simulink model "SimscapeCrane_StepInput"  (R2015a)
settings: Solver=ode15s  StartTime=0.0  StopTime=T  RelTol=1e-3
values from neighbouring files (symbols this model uses):
  filter_denominator = cell2mat(disc_filter.den)    [test.m]
  filter_numerator = cell2mat(disc_filter.num)    [test.m]
  H = B_big'*Q_big*B_big + R_big    [test.m]
  h_x = A_big'*Q_big*B_big    [test.m]
  m = 1    [test.m]
  N = 30    [test.m]
  Ts = 0.01    [test.m]
  Ts_mpc = 0.1    [test.m]
undefined symbols (not defined in the file or in its folder): MR, TxBreak, TxCoulomb, TxVisc, TyBreak, TyCoulomb, TzBreak, TzCoulomb, X, xRange, xZero, Y, yRange, yZero, Z, zRange, zZero
undefined symbols (not defined in the file): M, TorqueMultX, TorqueMultY, TorqueMultZ, TxTrans, TyTrans, TyVisc, TzTrans, TzVisc
libraries: sm_lib x146, fl_lib x62, nesl_utility x24, elec_lib x9, simulink x9, sm_double_wishbone_suspension_lib x4, aerolibtransform2 x1
(part 1 of 15)
settings Model: Creator=jsustare  LastModifiedBy=bkhusain
settings SolverCC: MaxConsecutiveMinStep=10  AutoInsertRateTranBlk=on  InsertRTBMode=Never (minimum delay)
settings DataIOCC: LimitDataPoints=off  SaveFormat=StructureWithTime
settings HardwareCC: ProdBitPerPointer=64  ProdLargestAtomicFloat=Float  ProdIntDivRoundTo=Zero  ProdEndianess=LittleEndian  ProdHWDeviceType=Specified
settings GRTTargetCC: GeneratePreprocessorConditionals=Use local settings

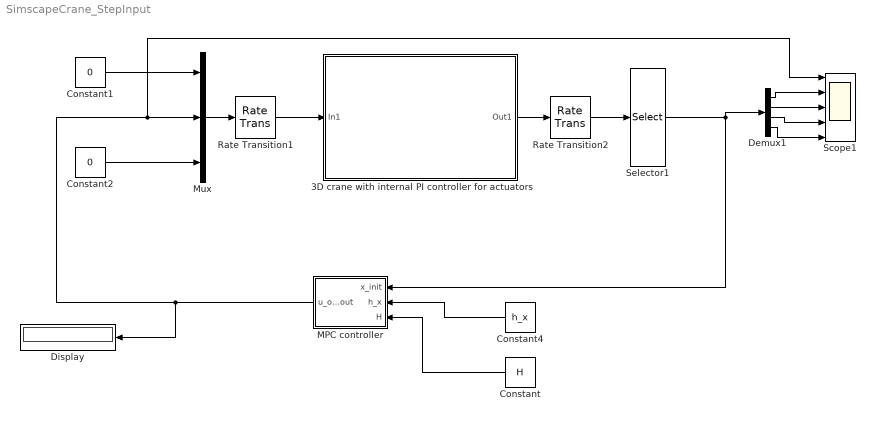
== system SimscapeCrane_StepInput ==
  " MPC controller" : MATLAB Function  TreatAsAtomicUnit=on
  3D crane with internal PI controller for actuators : Subsystem
  Constant : Constant  Value=H  SampleTime=Ts_mpc
  Constant1 : Constant  Value=0
  Constant2 : Constant  Value=0
  Constant4 : Constant  Value=h_x  SampleTime=Ts_mpc
  Demux1 : Demux
  Display : Display
  Mux : Mux  Inputs=3
  Rate Transition1 : RateTransition  Integrity=off  Deterministic=off  OutPortSampleTime=Ts
  Rate Transition2 : RateTransition  Integrity=off  Deterministic=off  OutPortSampleTime=Ts_mpc
  Scope1 : Scope  NumInputPorts=5
      settings: YMin=-0.0035~0.20025~-0.004~-0.0009~-0.00075  YMax=0.0005~0.202~0~0.0002~0.0015  SaveName=ScopeData5
  Selector1 : Selector  InputPortWidth=10  Indices=[3 4 9 10]
  wires:
  3D crane with internal PI controller for actuators/1(Out1) -> Rate Transition2/1
  Mux/1 -> Rate Transition1/1
  Constant1/1 -> Mux/1
  Constant2/1 -> Mux/3
  Selector1/1 -> Demux1/1, " MPC controller"/1(x_init)
  Constant/1 -> " MPC controller"/3(H)
  Constant4/1 -> " MPC controller"/2(h_x)
  " MPC controller"/1(u_opt_out) -> Display/1, Scope1/1, Mux/2
  Demux1/4 -> Scope1/5
  Demux1/3 -> Scope1/4
  Demux1/2 -> Scope1/3
  Demux1/1 -> Scope1/2
  Rate Transition1/1 -> 3D crane with internal PI controller for actuators/1(In1)
  Rate Transition2/1 -> Selector1/1
